simulink model "gm_RMS_computation"  (R2020a)
settings: Solver=FixedStepDiscrete  StartTime=0.0  StopTime=840000  RelTol=1e-3
undefined symbols (not defined in the file or in its folder): Newton, Raphson
libraries: hdlsllib x3, simulink x2
settings Model: FPTRunName=FPA_Reference  PacingRate=40  Creator=BuccelliLab  LastModifiedBy=diflo
settings SolverCC: AutoInsertRateTranBlk=on  MinimalZcImpactIntegration=on
settings DataIOCC: LimitDataPoints=on  SaveOutput=off  SaveTime=off  ReturnWorkspaceOutputs=off
settings OptimizationCC: BlockReduction=off  ConditionallyExecuteInputs=off  DefaultParameterBehavior=Inlined  LifeSpan=inf
settings DebuggingCC: SignalRangeChecking=warning  ReadBeforeWriteMsg=DisableAll  WriteAfterWriteMsg=DisableAll  WriteAfterReadMsg=DisableAll  AlgebraicLoopMsg=error  InheritedTsInSrcMsg=none  MultiTaskDSMMsg=none  SingleTaskRateTransMsg=error  ParameterDowncastMsg=warning  ParameterOverflowMsg=warning  AllowSymbolicDim=off  StrictBusMsg=ErrorOnBusTreatedAsVector  SFUnexpectedBacktrackingDiag=warning  SFNoUnconditionalDefaultTransitionDiag=warning  SFExecutionAtInitializationDiag=none  ArithmeticOperatorsInVariantConditions=warning
settings HardwareCC: ProdBitPerPointer=32  ProdBitPerSizeT=32  ProdBitPerPtrDiffT=32  ProdLargestAtomicFloat=None  ProdIntDivRoundTo=Undefined  ProdEndianess=Unspecified  ProdWordSize=32  ProdHWDeviceType=ASIC/FPGA->ASIC/FPGA  TargetBitPerPointer=64  TargetBitPerSizeT=64  TargetBitPerPtrDiffT=64  TargetLongLongMode=on  TargetIntDivRoundTo=Zero  TargetEndianess=LittleEndian  TargetWordSize=64  TargetHWDeviceType=Custom Processor->MATLAB Host Computer  ProdEqTarget=off
settings ModelReferenceCC: UpdateModelReferenceTargets=IfOutOfDate
settings SFSimCC: SFSimEcho=off  SimUseLocalCustomCode=off  CustomCodeUndefinedFunction=UseInterfaceOnly
settings RTWCC: RTWUseLocalCustomCode=off
settings CodeAppCC: StateflowObjectComments=on
settings GRTTargetCC: TargetLangStandard=C89/C90 (ANSI)
settings ConfigComp: CovScope=ReferencedModels  CovMetricSettings=dw  CovHtmlReporting=on  CovSaveCumulativeToWorkspaceVar=on  CovSaveSingleToWorkspaceVar=on  CovExternalEMLEnable=off  CovSFcnEnable=off

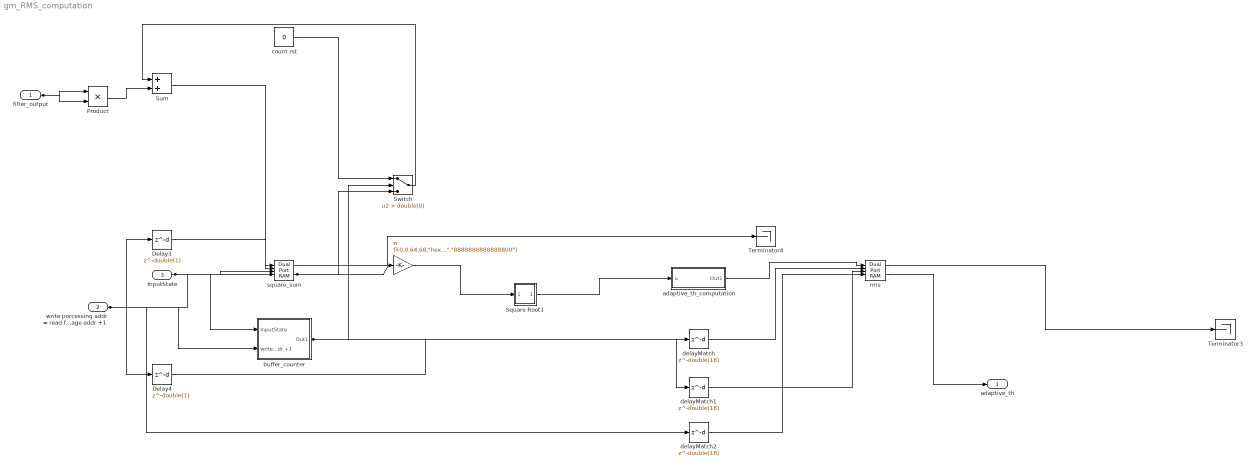
== system gm_RMS_computation ==
  filter_output : Inport  OutDataTypeStr=uint16  PortDimensions=1  SampleTime=1
  write porcessing addr = read from storage addr +1 : Inport  Port=2  OutDataTypeStr=fixdt(0, 9, 0)  PortDimensions=1  SampleTime=1
  InputState : Inport  Port=3  OutDataTypeStr=boolean  PortDimensions=1  SampleTime=1
  Delay3 : Delay  DelayLength=double(1)  InitialCondition=0  SampleTime=1
  Delay4 : Delay  DelayLength=double(1)  InitialCondition=0  SampleTime=1
  Product : Product  Inputs=**  OutDataTypeStr=uint32  SampleTime=1
  Square Root1 : Subsystem
  Sum : Sum  AccumDataTypeStr=fixdt(0, 65, 0)  OutDataTypeStr=fixdt(0, 64, 0)  SampleTime=1
  Switch : Switch  Criteria=u2 > Threshold  Threshold=double(0)  OutDataTypeStr=fixdt(0, 64, 0)  SampleTime=1
  Terminator3 : Terminator
  Terminator4 : Terminator
  adaptive_th_computation : Subsystem
  buffer_counter : Subsystem
  count rst : Constant  Value=0  OutDataTypeStr=fixdt(0, 64, 0)  SampleTime=1
  delayMatch : Delay  DelayLength=double(18)  InitialCondition=0  SampleTime=1
  delayMatch1 : Delay  DelayLength=double(18)  InitialCondition=0  SampleTime=1
  delayMatch2 : Delay  DelayLength=double(18)  InitialCondition=0  SampleTime=1
  n : Gain  Gain="fi(0,0,64,68,\"hex\",\"8888888888888800\")"  ParamDataTypeStr=fixdt(0, 64, 68)  OutDataTypeStr=fixdt(0, 40, 0)  SampleTime=1
  rms : hdlsllib/HDL RAMs/Dual Port RAM  ram_size=9
      settings: SourceProductBaseCode=SL
  square_sum : hdlsllib/HDL RAMs/Dual Port RAM  ram_size=9
      settings: SourceProductBaseCode=SL
  adaptive_th : Outport  OutDataTypeStr=uint16  PortDimensions=1  SampleTime=[1,0]
  wires:
  filter_output/1 -> Product/2, Product/1
  delayMatch2/1 -> rms/4
  InputState/1 -> buffer_counter/1(InputState), square_sum/3
  Delay3/1 -> square_sum/2
  delayMatch/1 -> rms/2
  Product/1 -> Sum/2
  Square Root1/1(Out1) -> adaptive_th_computation/1(u)
  adaptive_th_computation/1(Out1) -> rms/1
  delayMatch1/1 -> rms/3
  count rst/1 -> Switch/1
  n/1 -> Square Root1/1(In1)
  rms/1 -> Terminator3/1
  rms/2 -> adaptive_th/1
  square_sum/1 -> Terminator4/1
  square_sum/2 -> n/1, Switch/3
  Delay4/1 -> delayMatch/1
  buffer_counter/1(Out1) -> delayMatch1/1, Switch/2
  write porcessing addr = read from storage addr +1/1 -> delayMatch2/1, Delay4/1, Delay3/1, buffer_counter/2(write porcessing addr = read from storage addr +1), square_sum/4
  Sum/1 -> square_sum/1
  Switch/1 -> Sum/1

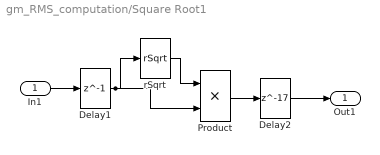
== system gm_RMS_computation/Square Root1 ==
  In1 : Inport
  Delay1 : Delay  DelayLength=1
  Delay2 : Delay  DelayLength=17
  Product : Product  OutDataTypeStr=uint16  SaturateOnIntegerOverflow=on
  rSqrt : Sqrt  Operator=rSqrt  OutDataTypeStr=fixdt(0,40,40)  RndMeth=Nearest  IntermediateResultsDataTypeStr=Inherit: Inherit from output  AlgorithmType=Newton-Raphson  SaturateOnIntegerOverflow=on
  Out1 : Outport
  wires:
  In1/1 -> Delay1/1
  Delay1/1 -> rSqrt/1, Product/2
  rSqrt/1 -> Product/1
  Product/1 -> Delay2/1
  Delay2/1 -> Out1/1

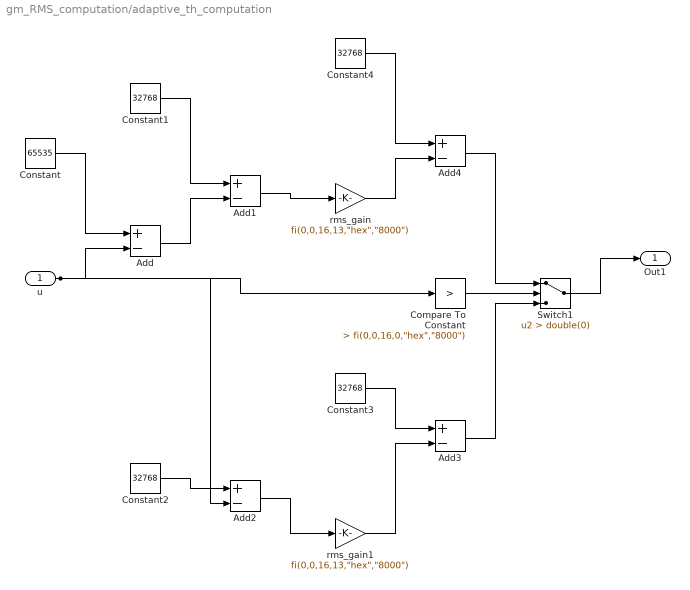
== system gm_RMS_computation/adaptive_th_computation ==
  u : Inport  OutDataTypeStr=uint16  PortDimensions=1  SampleTime=1
  Add{,1..4} (5 alike) : Sum  Inputs=+-  AccumDataTypeStr=uint16  OutDataTypeStr=uint16  SampleTime=1
  Compare To Constant : simulink/Logic and Bit Operations/Compare To Constant  relop=>  const="fi(0,0,16,0,\"hex\",\"8000\")"  OutDataTypeStr=boolean
  Constant : Constant  Value=65535  OutDataTypeStr=uint16  SampleTime=1
  Constant{1..4} (4 alike) : Constant  Value=32768  OutDataTypeStr=uint16  SampleTime=1
  Switch1 : Switch  Criteria=u2 > Threshold  Threshold=double(0)  OutDataTypeStr=uint16  SampleTime=1
  rms_gain : Gain  Gain="fi(0,0,16,13,\"hex\",\"8000\")"  ParamDataTypeStr=fixdt(0, 16, 13)  OutDataTypeStr=uint16  SampleTime=1
  rms_gain1 : Gain  Gain="fi(0,0,16,13,\"hex\",\"8000\")"  ParamDataTypeStr=fixdt(0, 16, 13)  OutDataTypeStr=uint16  SampleTime=1
  Out1 : Outport
  wires:
  Add/1 -> Add1/2
  Add1/1 -> rms_gain/1
  Add2/1 -> rms_gain1/1
  Add3/1 -> Switch1/3
  Add4/1 -> Switch1/1
  Compare To Constant/1 -> Switch1/2
  Constant/1 -> Add/1
  Constant1/1 -> Add1/1
  Constant2/1 -> Add2/1
  Constant3/1 -> Add3/1
  Constant4/1 -> Add4/1
  Switch1/1 -> Out1/1
  rms_gain/1 -> Add4/2
  rms_gain1/1 -> Add3/2
  u/1 -> Compare To Constant/1, Add2/2, Add/2

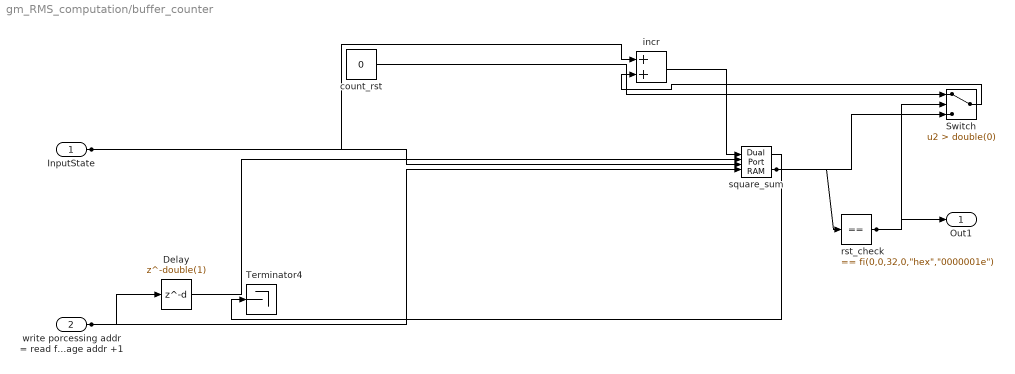
== system gm_RMS_computation/buffer_counter ==
  InputState : Inport  OutDataTypeStr=boolean  PortDimensions=1  SampleTime=1
  write porcessing addr = read from storage addr +1 : Inport  Port=2  OutDataTypeStr=fixdt(0, 9, 0)  PortDimensions=1  SampleTime=1
  Delay : Delay  DelayLength=double(1)  InitialCondition=0  SampleTime=1
  Switch : Switch  Criteria=u2 > Threshold  Threshold=double(0)  OutDataTypeStr=uint32  SampleTime=1
  Terminator4 : Terminator
  count_rst : Constant  Value=0  OutDataTypeStr=uint16  SampleTime=1
  incr : Sum  AccumDataTypeStr=uint32  OutDataTypeStr=uint32  SampleTime=1
  rst_check : simulink/Logic and Bit Operations/Compare To Constant  relop===  const="fi(0,0,32,0,\"hex\",\"0000001e\")"  OutDataTypeStr=boolean
  square_sum : hdlsllib/HDL RAMs/Dual Port RAM  ram_size=9
      settings: SourceProductBaseCode=SL
  Out1 : Outport
  wires:
  Delay/1 -> square_sum/2
  count_rst/1 -> Switch/1
  rst_check/1 -> Out1/1, Switch/2
  square_sum/1 -> Terminator4/1
  InputState/1 -> incr/1, square_sum/3
  write porcessing addr = read from storage addr +1/1 -> Delay/1, square_sum/4
  incr/1 -> square_sum/1
  Switch/1 -> incr/2
  square_sum/2 -> rst_check/1, Switch/3
